simulink model "tugasPSD (2)"  (R2018a)
settings: Solver=VariableStepAuto  StartTime=0.0  StopTime=2  RelTol=1e-3
values from neighbouring files (symbols this model uses):
  A = [0 1 0 0 0 0 0 0; b c f n o p d  e; 0 0 0 1 0 0 0 0; q r g h  0 0 s t; 0 0 0 0 0 1 0 0; u v 0 0 w x y z; 0 0 0 0 0 0 0 1; k m b3 b4 b2 b1 j i]    [12477_Untitled23.m]    (also in 12478_TUGAS2PSDuntitled.slx.m = [0 1 0 0 0 0 0 0; -(Kfs+Krs)/M -(Bf+Br)/M Kfs/M Bf/M Krs/M B; PSD (2).m = [0 1 0 0 0 0 0 0; (-(Kfs+Krs)/M) (-(Bf+Br)/M) (Kfs/M) (Bf/M))
  Ab = 4    [12477_Untitled23.m]    (also in 12478_TUGAS2PSDuntitled.slx.m; PSD (2).m)
  B = [0 0; 0 0; 0 0; (Kft/Mf) 0; 0 0; 0 (Kft/Mr); 0 0; 0 0;]    [12477_Untitled23.m]    (also in 12478_TUGAS2PSDuntitled.slx.m = [0 0; 0 0; 0 0; Kft/Mf 0; 0 0; 0 Kft/Mr; 0 0; 0 0;]; PSD (2).m = [0 0; 0 0; 0 0; (Kft/Mf) 0; 0 0; 0 (Kft/Mr); 0 0; 0 0])
  C = [1 0 0 0 0 0 0 0; 0 0 1 0 0 0 0 0; 0 0 0 0 1 0 0 0; 0 0 0 0 0 0 1 0;]    [12477_Untitled23.m]    (also in 12478_TUGAS2PSDuntitled.slx.m; PSD (2).m = [1 0 0 0 0 0 0 0; 0 0 1 0 0 0 0 0; 0 0 0 0 1 0 0 0; 0 0 0 0 )
  D = [0 0; 0 0; 0 0; 0 0;]    [12477_Untitled23.m]    (also in 12478_TUGAS2PSDuntitled.slx.m; PSD (2).m = [0 0; 0 0; 0 0; 0 0])
  L = 1    [12477_Untitled23.m]    (also in 12478_TUGAS2PSDuntitled.slx.m; PSD (2).m)
  Lf = 55    [12477_Untitled23.m]    (also in 12478_TUGAS2PSDuntitled.slx.m; PSD (2).m)
  Lr = 65    [12477_Untitled23.m]    (also in 12478_TUGAS2PSDuntitled.slx.m; PSD (2).m)
  V0 = 20    [PSD (2).m]
undefined symbols (not defined in the file or in its folder): D0
libraries: simulink_extras x1
settings Model: Creator=krisn  LastModifiedBy=krisn

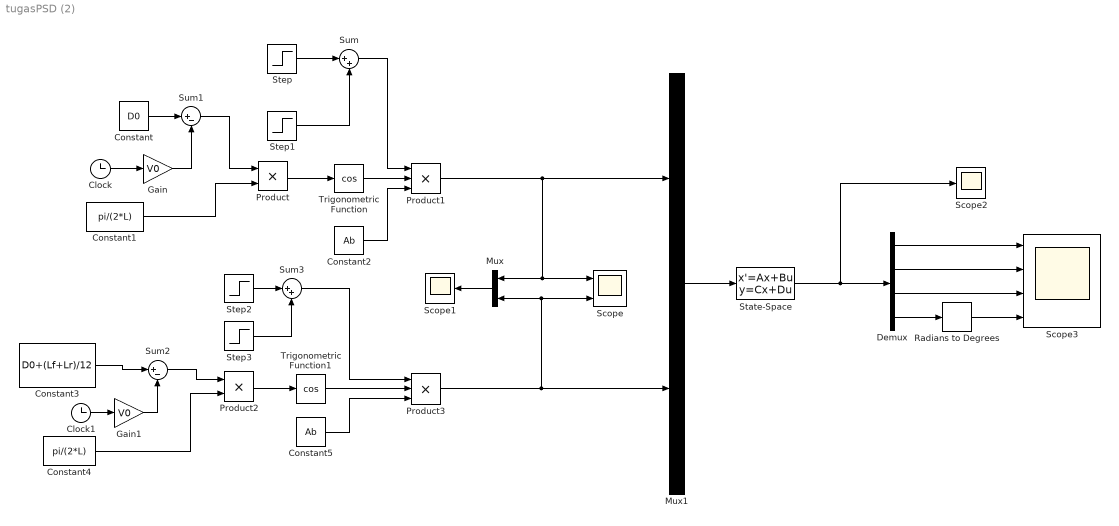
== system tugasPSD (2) ==
  Clock : Clock
  Clock1 : Clock
  Constant : Constant  Value=D0  OutMin=[1.75]  OutMax=[2.5]
  Constant1 : Constant  Value=pi/(2*L)
  Constant2 : Constant  Value=Ab
  Constant3 : Constant  Value=D0+(Lf+Lr)/12
  Constant4 : Constant  Value=pi/(2*L)
  Constant5 : Constant  Value=Ab
  Demux : Demux
  Gain : Gain  Gain=V0
  Gain1 : Gain  Gain=V0
  Mux : Mux  Inputs=2
  Mux1 : Mux  Inputs=2
  Product : Product
  Product1 : Product  Inputs=3
  Product2 : Product
  Product3 : Product  Inputs=3
  Radians to Degrees : simulink_extras/Transformations/Radians to Degrees
  Scope : Scope  NumInputPorts=2
  Scope1 : Scope
  Scope2 : Scope
  Scope3 : Scope  NumInputPorts=4
  State-Space : StateSpace  A=A  B=B  C=C  D=D  InitialCondition=0
  Step : Step  SampleTime=0
  Step1 : Step  Before=1  After=0  SampleTime=0
  Step2 : Step  SampleTime=0
  Step3 : Step  Before=1  After=0  SampleTime=0
  Sum : Sum  Inputs=|++
  Sum1 : Sum  Inputs=|+-
  Sum2 : Sum  Inputs=|+-
  Sum3 : Sum  Inputs=|++
  Trigonometric Function : Trigonometry  Operator=cos
  Trigonometric Function1 : Trigonometry  Operator=cos
  wires:
  Step/1 -> Sum/1
  Step1/1 -> Sum/2
  Clock/1 -> Gain/1
  Gain/1 -> Sum1/2
  Constant/1 -> Sum1/1
  Sum1/1 -> Product/1
  Constant1/1 -> Product/2
  Product/1 -> Trigonometric Function/1
  Trigonometric Function/1 -> Product1/2
  Constant2/1 -> Product1/3
  Sum/1 -> Product1/1
  Clock1/1 -> Gain1/1
  Constant3/1 -> Sum2/1
  Gain1/1 -> Sum2/2
  Sum2/1 -> Product2/1
  Constant4/1 -> Product2/2
  Product2/1 -> Trigonometric Function1/1
  Trigonometric Function1/1 -> Product3/2
  Step2/1 -> Sum3/1
  Step3/1 -> Sum3/2
  Sum3/1 -> Product3/1
  Constant5/1 -> Product3/3
  Product3/1 -> Mux/2, Scope/2, Mux1/2
  Product1/1 -> Scope/1, Mux/1, Mux1/1
  Mux/1 -> Scope1/1
  Mux1/1 -> State-Space/1
  State-Space/1 -> Demux/1, Scope2/1
  Demux/4 -> Radians to Degrees/1
  Radians to Degrees/1 -> Scope3/4
  Demux/3 -> Scope3/3
  Demux/2 -> Scope3/2
  Demux/1 -> Scope3/1
